simulink model "Cascade_FOC_BLDC_model"  (R2021b)
settings: Solver=ode15s  StartTime=0.0  StopTime=20.0  RelTol=1e-3
values from neighbouring files (symbols this model uses):
  Clarke = 2/3*[1 -1/2       -1/2 ... (first row only)    [motor_init.m]
  fourier_coeff_a = [ 0.08333    0.00000     0.00000 ... (first row only)    [motor_init.m]
  fourier_coeff_b = [-1.23020    0.60792     0.60792 ... (first row only)    [motor_init.m]
  J_m = 2.4059e-2    (= 0.024059)    [motor_init.m]
  J_m_inv = 1000*1/J_m    (= 41564.487302)    [motor_init.m]
  K_e = 0.052    [motor_init.m]
  L_m = 8.97e-6    (= 8.97e-06)    [motor_init.m]
  n_pole_pairs = n_poles/2    (= 7)    [motor_init.m]
  psi_m = 4.88e-3    (= 0.00488)    [motor_init.m]
  R_m = 19.00e-3    (= 0.019)    [motor_init.m]
settings Model: PacingRate=11  Creator=Sølve  LastModifiedBy=Sølve

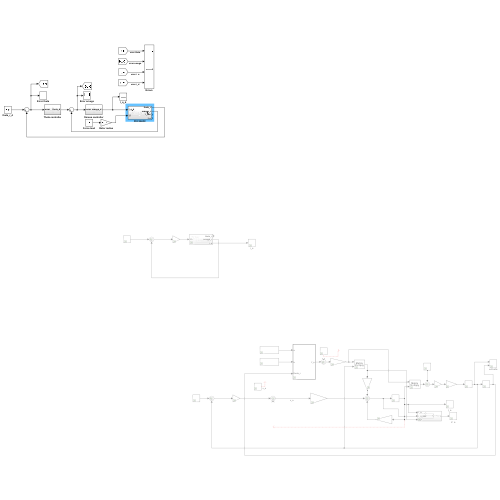
[thumbnail: Simulink's stored preview of the top-level diagram]
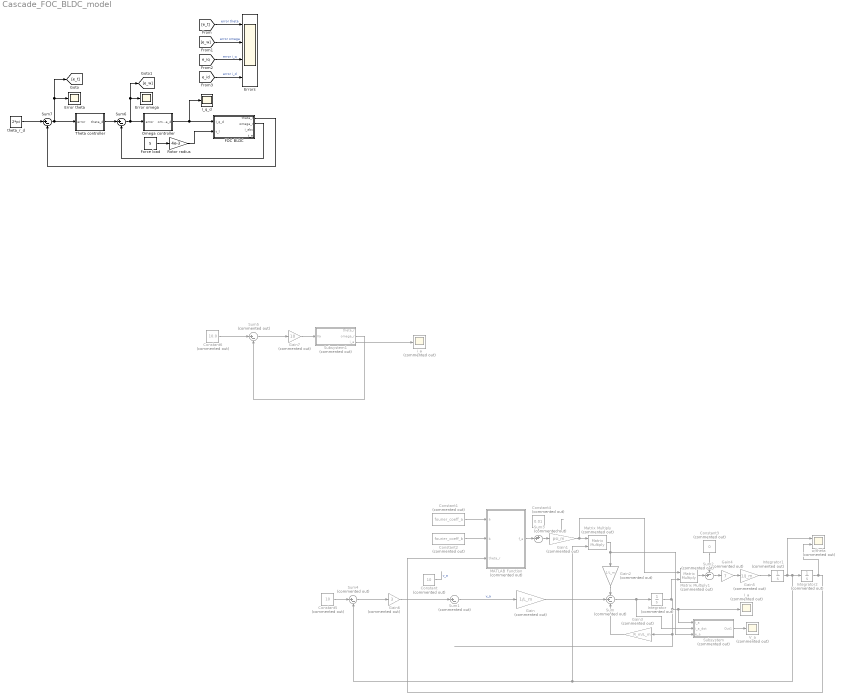
== system Cascade_FOC_BLDC_model ==
  Constant : Constant  Commented=on  Value=10
  Constant1 : Constant  Commented=on  Value=fourier_coeff_a
  Constant2 : Constant  Commented=on  Value=fourier_coeff_b
  Constant3 : Constant  Commented=on  Value=0
  Constant4 : Constant  Commented=on  Value=0.01
  Constant5 : Constant  Commented=on  Value=10
  Constant6 : Constant  Commented=on  Value=10.0
  Error omega : Scope
  Error theta : Scope
  Errors : Scope  NumInputPorts=4
  FOC BLDC : Subsystem
  Force load : Constant  Value=5
  Gain : Gain  Commented=on  Gain=1/L_m
  Gain1 : Gain  Commented=on  Gain=psi_m
  Gain2 : Gain  Commented=on  Gain=1/L_m
  Gain3 : Gain  Commented=on  Gain=R_m/L_m
  Gain4 : Gain  Commented=on  Gain=7
  Gain5 : Gain  Commented=on  Gain=1/J_m
  Gain6 : Gain  Commented=on  Gain=3
  Gain7 : Gain  Commented=on  Gain=10
  I_a : Scope  Commented=on
  I_q_d : Scope
  Integrator : Integrator  Commented=on
  Integrator1 : Integrator  Commented=on
  Integrator2 : Integrator  Commented=on  InitialCondition=pi/2
  MATLAB Function : MATLAB Function  Commented=on  TreatAsAtomicUnit=on
  Matrix Multiply : Product  Commented=on  Multiplication=Matrix(*)
  Matrix Multiply1 : Product  Commented=on  Multiplication=Matrix(*)
  Omega controller : Subsystem
  Rotor radius : Gain  Gain=4e-3
  Subsystem : Subsystem  Commented=on
  Subsystem1 : Subsystem  Commented=on
  Sum : Sum  Commented=on  Inputs=-+-
  Sum1 : Sum  Commented=on  Inputs=|+-
  Sum2 : Sum  Commented=on  Inputs=-+|
  Sum3 : Sum  Commented=on  Inputs=++|
  Sum4 : Sum  Commented=on  Inputs=|+-
  Sum5 : Sum  Commented=on  Inputs=|+-
  Sum6 : Sum  Inputs=|+-
  Sum7 : Sum  Inputs=|+-
  Theta controller : Subsystem
  V_a : Scope  Commented=on
  i_a : Scope  Commented=on
  theta_r_d : Constant  Value=2*pi
  w/theta : Scope  Commented=on  NumInputPorts=2
  wires:
  Sum1/1 -> Gain/1  "v_a"
  Constant1/1 -> MATLAB Function/1(a)
  Constant2/1 -> MATLAB Function/2(b)
  MATLAB Function/1(f_a) -> Sum3/2
  Gain1/1 -> Matrix Multiply1/1, Matrix Multiply/1
  Gain/1 -> Sum/2
  Matrix Multiply/1 -> Subsystem/3(e_a), Gain2/1
  Gain2/1 -> Sum/1
  Sum/1 -> Subsystem/2(i_a_dot), Integrator/1
  Integrator/1 -> Subsystem/1(i_a), I_a/1, Gain3/1, Matrix Multiply1/2
  Gain3/1 -> Sum/3
  Constant/1 -> ?  "v_a"
  Matrix Multiply1/1 -> Sum2/2
  Constant3/1 -> Sum2/1
  Sum2/1 -> Gain4/1
  Gain4/1 -> Gain5/1
  Gain5/1 -> Integrator1/1
  Integrator2/1 -> w/theta/2, MATLAB Function/3(theta_r)
  Integrator1/1 -> w/theta/1, Sum4/2, Matrix Multiply/2, Integrator2/1
  Subsystem/1(Out1) -> V_a/1
  Sum3/1 -> Gain1/1
  Constant4/1 -> ?
  Constant5/1 -> Sum4/1
  Sum4/1 -> Gain6/1
  Gain6/1 -> Sum1/1
  Constant6/1 -> Sum5/1
  Sum5/1 -> Gain7/1
  Subsystem1/3(i_a) -> i_a/1
  Gain7/1 -> Subsystem1/1(Va)
  Subsystem1/2(omega_r) -> Sum5/2
  Sum6/1 -> Omega controller/1(error), Error omega/1, [e_w]
  Omega controller/1(omega_d) -> I_q_d/1, FOC BLDC/1(I_q_d)
  FOC BLDC/2(omega_r) -> Sum6/2
  Force load/1 -> Rotor radius/1
  Sum7/1 -> Theta controller/1(error), [e_t], Error theta/1
  Theta controller/1(theta_d) -> Sum6/1
  FOC BLDC/1(theta_r) -> Sum7/2
  theta_r_d/1 -> Sum7/1
  [e_t] -> Errors/1  "error theta"
  [e_w] -> Errors/2  "error omega"
  [e_iq] -> Errors/3  "error i_q"
  [e_id] -> Errors/4  "error i_d"
  Rotor radius/1 -> FOC BLDC/2(t_l)

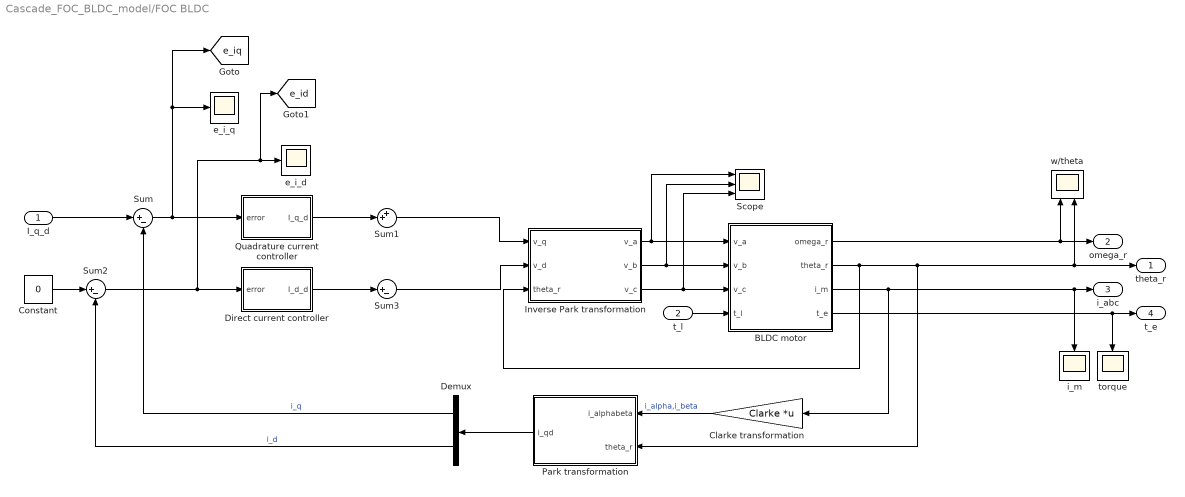
== system Cascade_FOC_BLDC_model/FOC BLDC ==
  I_q_d : Inport
  t_l : Inport  Port=2
  BLDC motor : Subsystem
  Clarke transformation : Gain  Gain=Clarke  Multiplication=Matrix(K*u) (u vector)
  Constant : Constant  Value=0
  Demux : Demux  Outputs=2
  Direct current controller : Subsystem
  Inverse Park transformation : MATLAB Function  TreatAsAtomicUnit=on
  Park transformation : MATLAB Function  TreatAsAtomicUnit=on
  Quadrature current controller : Subsystem
  Scope : Scope  NumInputPorts=3
  Sum : Sum  Inputs=|+-
  Sum1 : Sum  Inputs=++|
  Sum2 : Sum  Inputs=|+-
  Sum3 : Sum  Inputs=|+-
  e_i_d : Scope
  e_i_q : Scope
  i_m : Scope
  torque : Scope
  w/theta : Scope  NumInputPorts=2
  theta_r : Outport
  omega_r : Outport  Port=2
  i_abc : Outport  Port=3
  t_e : Outport  Port=4
  tag scope: e_id=global, e_iq=global
  wires:
  Sum/1 -> Quadrature current controller/1(error), [e_iq], e_i_q/1
  Quadrature current controller/1(I_q_d) -> Sum1/2
  Constant/1 -> Sum2/1
  Sum2/1 -> Direct current controller/1(error), [e_id], e_i_d/1
  Direct current controller/1(I_d_d) -> Sum3/1
  Sum1/1 -> Inverse Park transformation/1(v_q)
  Sum3/1 -> Inverse Park transformation/2(v_d)
  Inverse Park transformation/1(v_a) -> Scope/1, BLDC motor/1(v_a)
  Inverse Park transformation/2(v_b) -> Scope/2, BLDC motor/2(v_b)
  Inverse Park transformation/3(v_c) -> Scope/3, BLDC motor/3(v_c)
  t_l/1 -> BLDC motor/4(t_l)
  BLDC motor/1(omega_r) -> omega_r/1, w/theta/1
  Clarke transformation/1 -> Park transformation/1(i_alphabeta)  "i_alpha,i_beta"
  BLDC motor/2(theta_r) -> Park transformation/2(theta_r), theta_r/1, w/theta/2, Inverse Park transformation/3(theta_r)
  Park transformation/1(i_qd) -> Demux/1
  Demux/1 -> Sum/2  "i_q"
  Demux/2 -> Sum2/2  "i_d"
  BLDC motor/3(i_m) -> i_m/1, i_abc/1, Clarke transformation/1
  BLDC motor/4(t_e) -> torque/1, t_e/1
  I_q_d/1 -> Sum/1

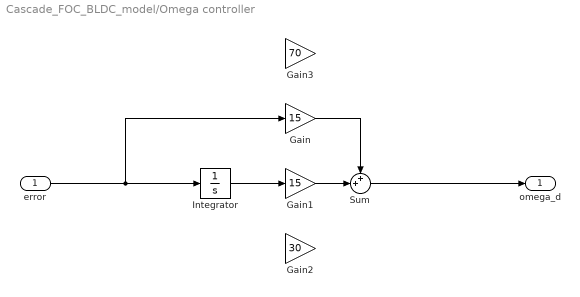
== system Cascade_FOC_BLDC_model/Omega controller ==
  error : Inport
  Gain : Gain  Gain=15
  Gain1 : Gain  Gain=15
  Gain2 : Gain  Gain=30
  Gain3 : Gain  Gain=70
  Integrator : Integrator
  Sum : Sum  Inputs=++|
  omega_d : Outport
  wires:
  Sum/1 -> omega_d/1
  Gain/1 -> Sum/1
  Gain1/1 -> Sum/2
  Integrator/1 -> Gain1/1
  error/1 -> Integrator/1, Gain/1

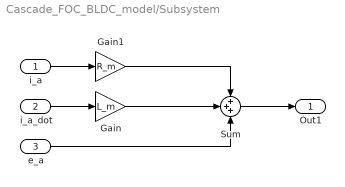
== system Cascade_FOC_BLDC_model/Subsystem ==
  i_a : Inport
  i_a_dot : Inport  Port=2
  e_a : Inport  Port=3
  Gain : Gain  Gain=L_m
  Gain1 : Gain  Gain=R_m
  Sum : Sum  Inputs=+++
  Out1 : Outport
  wires:
  i_a_dot/1 -> Gain/1
  i_a/1 -> Gain1/1
  Gain1/1 -> Sum/1
  Gain/1 -> Sum/2
  e_a/1 -> Sum/3
  Sum/1 -> Out1/1

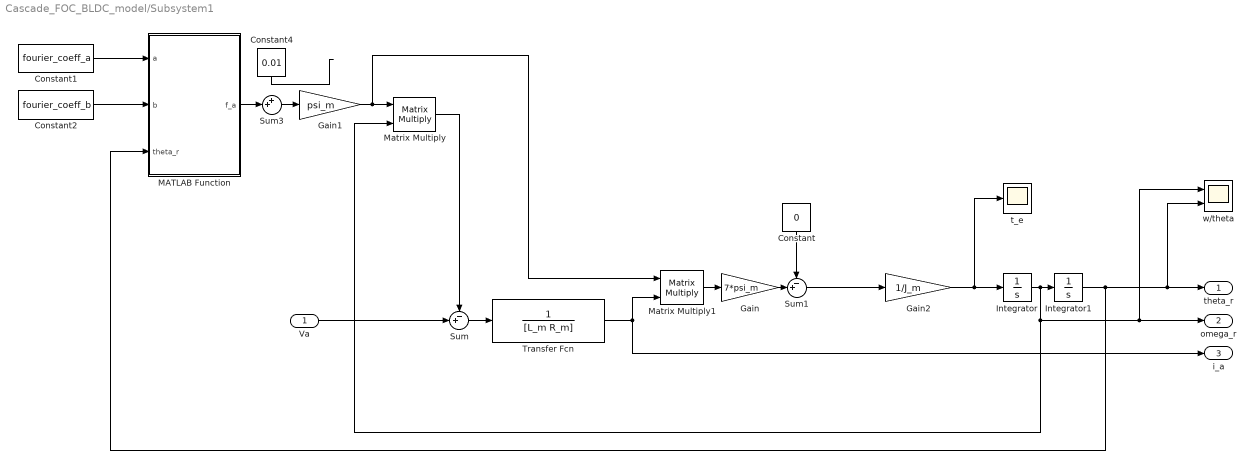
== system Cascade_FOC_BLDC_model/Subsystem1 ==
  Va : Inport
  Constant : Constant  Value=0
  Constant1 : Constant  Value=fourier_coeff_a
  Constant2 : Constant  Value=fourier_coeff_b
  Constant4 : Constant  Value=0.01
  Gain : Gain  Gain=7*psi_m
  Gain1 : Gain  Gain=psi_m
  Gain2 : Gain  Gain=1/J_m
  Integrator : Integrator
  Integrator1 : Integrator  InitialCondition=pi/2
  MATLAB Function : MATLAB Function  TreatAsAtomicUnit=on
  Matrix Multiply : Product  Multiplication=Matrix(*)
  Matrix Multiply1 : Product  Multiplication=Matrix(*)
  Sum : Sum  Inputs=-+|
  Sum1 : Sum  Inputs=-+|
  Sum3 : Sum  Inputs=++|
  Transfer Fcn : TransferFcn  Denominator=[L_m R_m]
  t_e : Scope
  w/theta : Scope  NumInputPorts=2
  theta_r : Outport
  omega_r : Outport  Port=2
  i_a : Outport  Port=3
  wires:
  Constant4/1 -> ?
  Sum3/1 -> Gain1/1
  MATLAB Function/1(f_a) -> Sum3/2
  Constant2/1 -> MATLAB Function/2(b)
  Constant1/1 -> MATLAB Function/1(a)
  Gain1/1 -> Matrix Multiply1/1, Matrix Multiply/1
  Integrator/1 -> w/theta/1, omega_r/1, Matrix Multiply/2, Integrator1/1
  Matrix Multiply/1 -> Sum/1
  Va/1 -> Sum/2
  Sum/1 -> Transfer Fcn/1
  Transfer Fcn/1 -> i_a/1, Matrix Multiply1/2
  Matrix Multiply1/1 -> Gain/1
  Gain/1 -> Sum1/2
  Constant/1 -> Sum1/1
  Sum1/1 -> Gain2/1
  Integrator1/1 -> w/theta/2, theta_r/1, MATLAB Function/3(theta_r)
  Gain2/1 -> t_e/1, Integrator/1

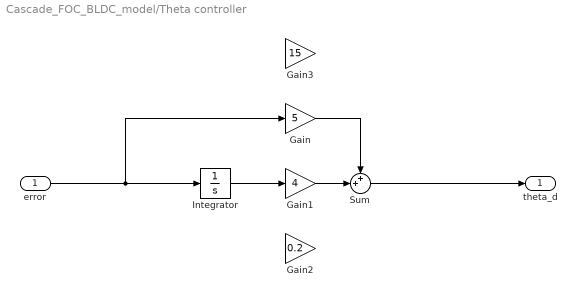
== system Cascade_FOC_BLDC_model/Theta controller ==
  error : Inport
  Gain : Gain  Gain=5
  Gain1 : Gain  Gain=4
  Gain2 : Gain  Gain=0.2
  Gain3 : Gain  Gain=15
  Integrator : Integrator
  Sum : Sum  Inputs=++|
  theta_d : Outport
  wires:
  error/1 -> Gain/1, Integrator/1
  Integrator/1 -> Gain1/1
  Gain1/1 -> Sum/2
  Gain/1 -> Sum/1
  Sum/1 -> theta_d/1

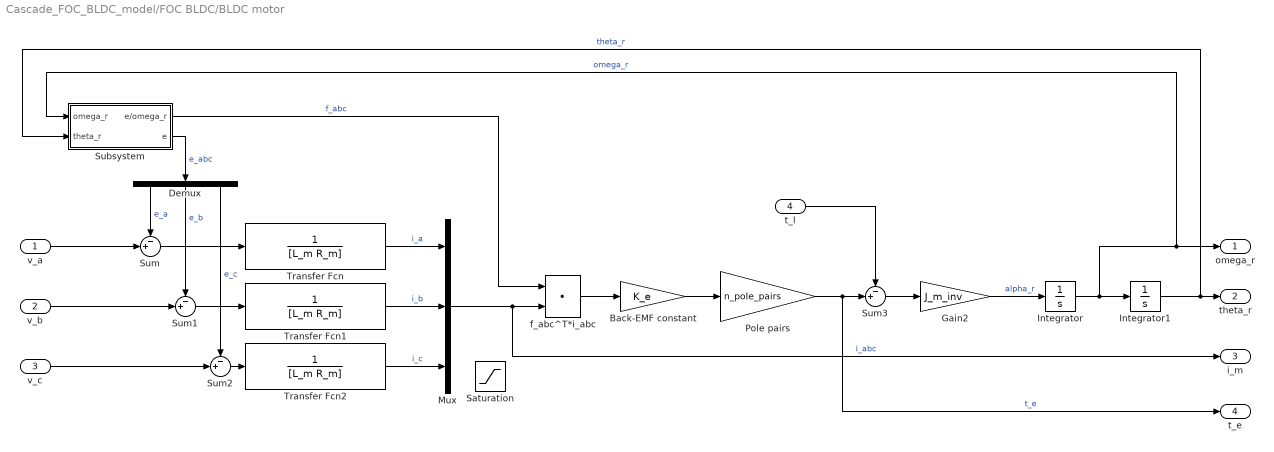
== system Cascade_FOC_BLDC_model/FOC BLDC/BLDC motor ==
  v_a : Inport
  v_b : Inport  Port=2
  v_c : Inport  Port=3
  t_l : Inport  Port=4
  Back-EMF constant : Gain  Gain=K_e
  Demux : Demux  Outputs=3
  Gain2 : Gain  Gain=J_m_inv
  Integrator : Integrator  InitialCondition=0.001
  Integrator1 : Integrator
  Mux : Mux  Inputs=3
  Pole pairs : Gain  Gain=n_pole_pairs
  Saturation : Saturate  UpperLimit=20  LowerLimit=20
  Subsystem : Subsystem
  Sum{,1..3} (4 alike) : Sum  Inputs=-+|
  Transfer Fcn : TransferFcn  Denominator=[L_m R_m]
  Transfer Fcn1 : TransferFcn  Denominator=[L_m R_m]
  Transfer Fcn2 : TransferFcn  Denominator=[L_m R_m]
  f_abc^T*i_abc : DotProduct  InputSameDT=on  OutDataTypeStr=Inherit: Inherit via internal rule
  omega_r : Outport
  theta_r : Outport  Port=2
  i_m : Outport  Port=3
  t_e : Outport  Port=4
  wires:
  v_a/1 -> Sum/2
  v_b/1 -> Sum1/2
  v_c/1 -> Sum2/2
  Demux/1 -> Sum/1  "e_a"
  Demux/2 -> Sum1/1  "e_b"
  Demux/3 -> Sum2/1  "e_c"
  Subsystem/2(e) -> Demux/1  "e_abc"
  Sum/1 -> Transfer Fcn/1
  Sum1/1 -> Transfer Fcn1/1
  Sum2/1 -> Transfer Fcn2/1
  Transfer Fcn2/1 -> Mux/3  "i_c"
  Transfer Fcn1/1 -> Mux/2  "i_b"
  Transfer Fcn/1 -> Mux/1  "i_a"
  Subsystem/1(e/omega_r) -> f_abc^T*i_abc/1  "f_abc"
  Sum3/1 -> Gain2/1
  f_abc^T*i_abc/1 -> Back-EMF constant/1
  Back-EMF constant/1 -> Pole pairs/1
  t_l/1 -> Sum3/1
  Gain2/1 -> Integrator/1  "alpha_r"
  Integrator/1 -> Subsystem/1(omega_r), omega_r/1, Integrator1/1  "omega_r"
  Integrator1/1 -> theta_r/1, Subsystem/2(theta_r)  "theta_r"
  Pole pairs/1 -> t_e/1, Sum3/2  "t_e"
  Mux/1 -> f_abc^T*i_abc/2, i_m/1  "i_abc"

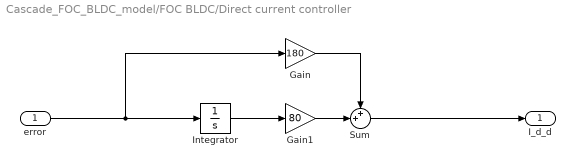
== system Cascade_FOC_BLDC_model/FOC BLDC/Direct current controller ==
  error : Inport
  Gain : Gain  Gain=180
  Gain1 : Gain  Gain=80
  Integrator : Integrator
  Sum : Sum  Inputs=++|
  I_d_d : Outport
  wires:
  error/1 -> Gain/1, Integrator/1
  Integrator/1 -> Gain1/1
  Gain1/1 -> Sum/2
  Gain/1 -> Sum/1
  Sum/1 -> I_d_d/1

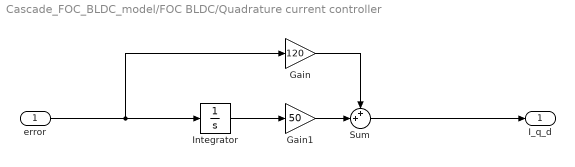
== system Cascade_FOC_BLDC_model/FOC BLDC/Quadrature current controller ==
  error : Inport
  Gain : Gain  Gain=120
  Gain1 : Gain  Gain=50
  Integrator : Integrator
  Sum : Sum  Inputs=++|
  I_q_d : Outport
  wires:
  Sum/1 -> I_q_d/1
  Gain/1 -> Sum/1
  Gain1/1 -> Sum/2
  Integrator/1 -> Gain1/1
  error/1 -> Integrator/1, Gain/1

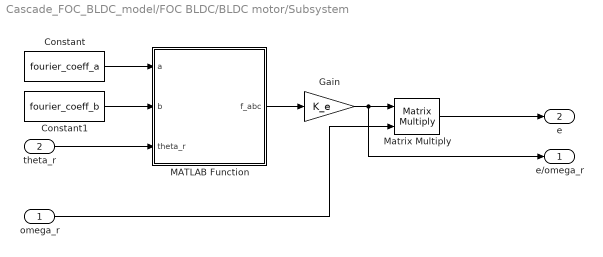
== system Cascade_FOC_BLDC_model/FOC BLDC/BLDC motor/Subsystem ==
  omega_r : Inport
  theta_r : Inport  Port=2
  Constant : Constant  Value=fourier_coeff_a
  Constant1 : Constant  Value=fourier_coeff_b
  Gain : Gain  Gain=K_e
  MATLAB Function : MATLAB Function  TreatAsAtomicUnit=on
  Matrix Multiply : Product  Multiplication=Matrix(*)
  e/omega_r : Outport
  e : Outport  Port=2
  wires:
  theta_r/1 -> MATLAB Function/3(theta_r)
  Constant/1 -> MATLAB Function/1(a)
  Constant1/1 -> MATLAB Function/2(b)
  MATLAB Function/1(f_abc) -> Gain/1
  Gain/1 -> e/omega_r/1, Matrix Multiply/1
  omega_r/1 -> Matrix Multiply/2
  Matrix Multiply/1 -> e/1

== matlab function Cascade_FOC_BLDC_model/Subsystem1/MATLAB Function ==
  data: a input; f_a output; b input; theta_r input
function f_a  = normalized_back_EMF(a,b,theta_r)
sa = 0;
ca = 0;

n = size(a,1);

for i = 1:2:n
    sa = sa + b(i,1)*sin(i*theta_r);
end
f_a = ca+sa;

% f_abc = [f_a;f_b;f_c];

== matlab function Cascade_FOC_BLDC_model/MATLAB Function ==
  data: a input; f_a output; b input; theta_r input
function f_a  = normalized_back_EMF(a,b,theta_r)
sa = 0;
ca = 0;

n = size(a,1);

for i = 1:2:n
    sa = sa + b(i,1)*sin(i*theta_r);
end
f_a = ca+sa;

% f_abc = [f_a;f_b;f_c];

== matlab function Cascade_FOC_BLDC_model/FOC BLDC/Inverse Park transformation ==
  data: v_q input; v_d input; v_a output; theta_r input; v_b output; v_c output
function [v_a, v_b, v_c] = inverse_park(v_q, v_d, theta_r)
Park_inv = [cos(theta_r)          -sin(theta_r);
            cos(theta_r - 2*pi/3) -sin(theta_r - 2*pi/3);
            cos(theta_r + 2*pi/3) -sin(theta_r + 2*pi/3)];

v_abc = Park_inv*[v_d;v_q];

v_a = v_abc(1);
v_b = v_abc(2);
v_c = v_abc(3);

== matlab function Cascade_FOC_BLDC_model/FOC BLDC/BLDC motor/Subsystem/MATLAB Function ==
  data: a input; f_abc output; b input; theta_r input
function f_abc  = normalized_back_EMF(a,b,theta_r)
sa = 0;
sb = 0;
sc = 0;
ca = 0;
cb = 0;
cc = 0;
n = size(a,1);

for i = 1:n
%     ca = ca + a(i,1)*cos((i-1)*theta_r);
    cb = cb + a(i,2)*cos((i-1)*theta_r);
    cc = cc + a(i,3)*cos((i-1)*theta_r); 
end
for i = 1:2:n
    sa = sa + b(i,1)*sin(i*theta_r);
    sb = sb + b(i,2)*sin(i*theta_r);
    sc = sc + b(i,3)*sin(i*theta_r);
end
f_a = ca+sa;
f_b = cb+sb;
f_c = cc+sc;

f_abc = [f_a;f_b;f_c];

== matlab function Cascade_FOC_BLDC_model/FOC BLDC/Park transformation ==
  data: i_alphabeta input; i_qd output; theta_r input
function i_qd = park(i_alphabeta, theta_r)
Park = [-sin(theta_r) cos(theta_r);
         cos(theta_r) sin(theta_r)];
i_qd = Park*i_alphabeta;
